simulink model "Feedback_effectOn_SteadyStateError"  (R2023b)
settings: Solver=VariableStepAuto  StartTime=0.0  StopTime=10.0  RelTol=1e-3
settings Model: Creator=reemb  LastModifiedBy=reemb

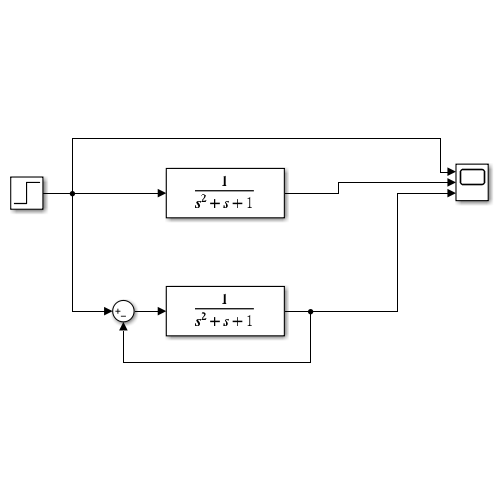
[thumbnail: Simulink's stored preview of the top-level diagram]
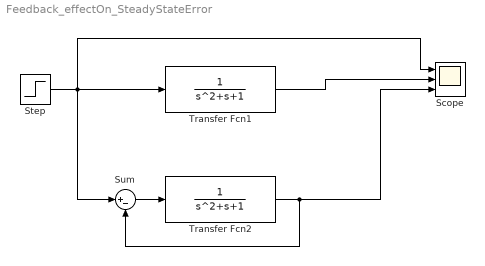
== system Feedback_effectOn_SteadyStateError ==
  Scope : Scope  NumInputPorts=3
  Step : Step  SampleTime=0
  Sum : Sum  Inputs=|+-
  Transfer Fcn1 : TransferFcn  Denominator=[1 1 1]
  Transfer Fcn2 : TransferFcn  Denominator=[1 1 1]
  wires:
  Transfer Fcn1/1 -> Scope/2
  Transfer Fcn2/1 -> Scope/3, Sum/2
  Sum/1 -> Transfer Fcn2/1
  Step/1 -> Sum/1, Scope/1, Transfer Fcn1/1
